simulink model "ex2"  (R2015a)
settings: Solver=ode45  StartTime=0.0  StopTime=10  RelTol=1e-3
values from neighbouring files (symbols this model uses):
  A = gss.a    [ex2.m]
  B = gss.b    [ex2.m]
  C = gss.c    [ex2.m]
  D = gss.d    [ex2.m]
  K = place(Aa,Ba,[-4 -5 -7])    [ex2.m]
libraries: simulink x1
settings Model: Creator=Kostas  LastModifiedBy=Xrisostomos

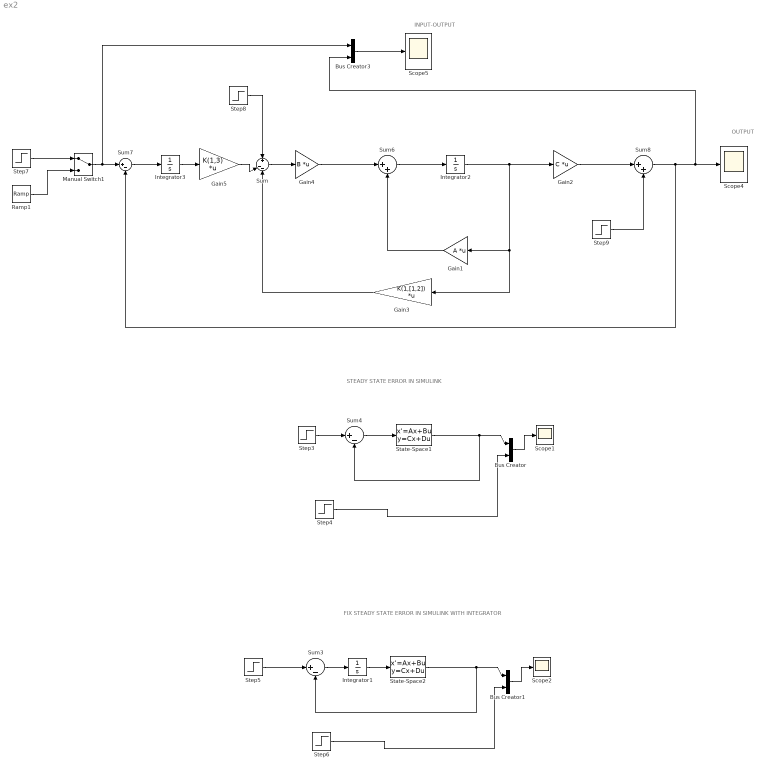
== system ex2 ==
  note: OUTPUT
  note: INPUT-OUTPUT
  note: STEADY STATE ERROR IN SIMULINK
  note: FIX STEADY STATE ERROR IN SIMULINK WITH INTEGRATOR
  Bus Creator : BusCreator  Inputs=2
  Bus Creator1 : BusCreator  Inputs=2
  Bus Creator3 : BusCreator  Inputs=2
  Gain1 : Gain  Gain=A  Multiplication=Matrix(K*u)
  Gain2 : Gain  Gain=C  Multiplication=Matrix(K*u)
  Gain3 : Gain  Gain=K(1,[1,2])  Multiplication=Matrix(K*u)
  Gain4 : Gain  Gain=B  Multiplication=Matrix(K*u)
  Gain5 : Gain  Gain=K(1,3)  Multiplication=Matrix(K*u)
  Integrator1 : Integrator
  Integrator2 : Integrator
  Integrator3 : Integrator
  Manual Switch1 : ManualSwitch
  Ramp1 : simulink/Sources/Ramp  slope=1  start=0  X0=0
  Scope{1..2,4..5} (4 alike) : Scope
      Scope2 settings: SaveName=ScopeData2
      Scope4 settings: TimeRange=2  YMin=0  YMax=0.0004  SaveName=ScopeData4
      Scope5 settings: TimeRange=2  YMin=0  YMax=0.0004  SaveName=ScopeData5
  State-Space1 : StateSpace  A=A  B=B  C=C  D=D  X0=0
  State-Space2 : StateSpace  A=A  B=B  C=C  D=D  X0=0
  Step3 : Step  Time=0  SampleTime=0
  Step4 : Step  Time=4  After=0.5  SampleTime=0
  Step5 : Step  Time=0  SampleTime=0
  Step6 : Step  Time=4  SampleTime=0
  Step7 : Step  SampleTime=0
  Step8 : Step  Time=4  After=0.5  SampleTime=0
  Step9 : Step  Time=8  After=0.5  SampleTime=0
  Sum : Sum  Inputs=+|--
  Sum3 : Sum  Inputs=|+-
  Sum4 : Sum  Inputs=|+-
  Sum6 : Sum  Inputs=|++
  Sum7 : Sum  Inputs=|+-
  Sum8 : Sum  Inputs=|++
  wires:
  Sum4/1 -> State-Space1/1
  State-Space1/1 -> Sum4/2, Bus Creator/1
  Step3/1 -> Sum4/1
  Step4/1 -> Bus Creator/2
  Bus Creator/1 -> Scope1/1
  State-Space2/1 -> Sum3/2, Bus Creator1/1
  Step6/1 -> Bus Creator1/2
  Bus Creator1/1 -> Scope2/1
  Step5/1 -> Sum3/1
  Sum3/1 -> Integrator1/1
  Integrator1/1 -> State-Space2/1
  Sum6/1 -> Integrator2/1
  Integrator2/1 -> Gain3/1, Gain1/1, Gain2/1
  Gain3/1 -> Sum/3
  Gain1/1 -> Sum6/2
  Gain4/1 -> Sum6/1
  Sum/1 -> Gain4/1
  Gain5/1 -> Sum/2
  Integrator3/1 -> Gain5/1
  Sum7/1 -> Integrator3/1
  Step8/1 -> Sum/1
  Gain2/1 -> Sum8/1
  Step9/1 -> Sum8/2
  Sum8/1 -> Bus Creator3/2, Scope4/1, Sum7/2
  Ramp1/1 -> Manual Switch1/2
  Step7/1 -> Manual Switch1/1
  Manual Switch1/1 -> Bus Creator3/1, Sum7/1
  Bus Creator3/1 -> Scope5/1
